simulink model "Models"  (R2022a)
settings: Solver=VariableStepAuto  StartTime=0.0  StopTime=15  RelTol=1e-6
settings Model: Creator=derekyu  LastModifiedBy=derekyu

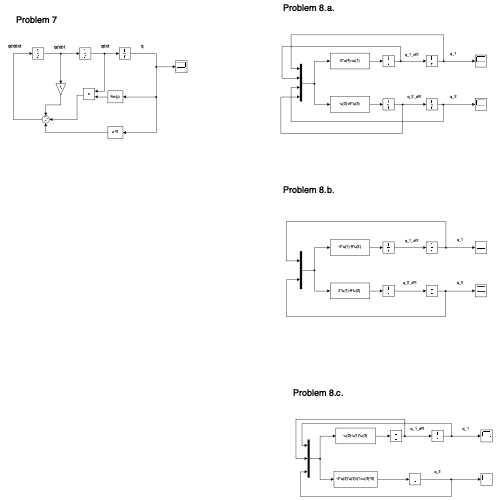
[thumbnail: Simulink's stored preview of the top-level diagram]
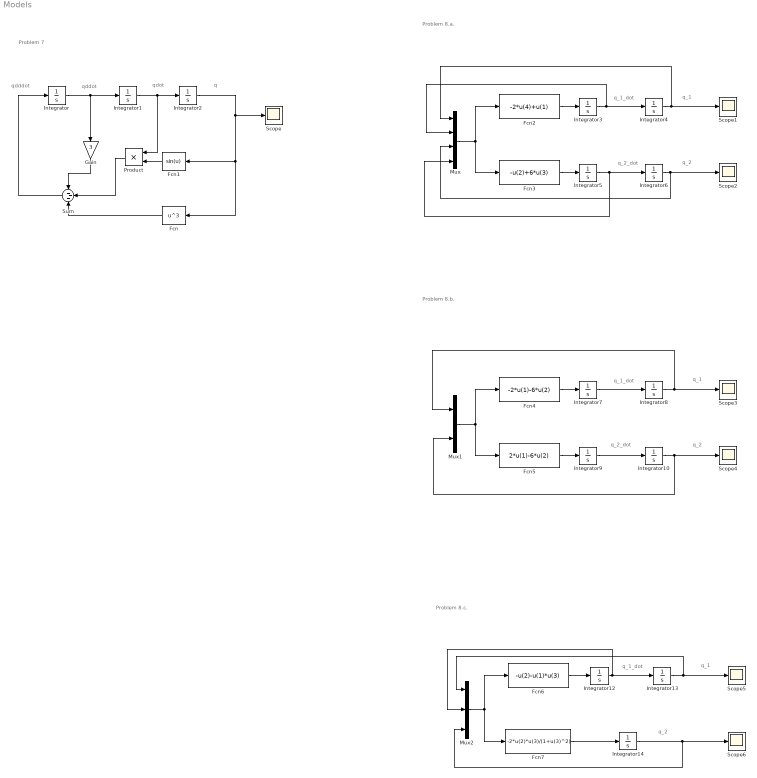
== system Models ==
  note: q_1_dot
  note: qdddot
  note: Problem 7
  note: qddot
  note: qdot
  note: q
  note: Problem 8.a.
  note: q_1
  note: q_2_dot
  note: q_2
  note: Problem 8.b.
  note: q_2
  note: q_1
  note: q_2_dot
  note: q_1_dot
  note: Problem 8.c.
  note: q_2
  note: q_1
  note: q_1_dot
  Fcn : Fcn  Expr=u^3
  Fcn1 : Fcn  Expr=sin(u)
  Fcn2 : Fcn  Expr=-2*u(4)+u(1)
  Fcn3 : Fcn  Expr=-u(2)+6*u(3)
  Fcn4 : Fcn  Expr=-2*u(1)-6*u(2)
  Fcn5 : Fcn  Expr=2*u(1)-6*u(2)
  Fcn6 : Fcn  Expr=-u(2)-u(1)*u(3)
  Fcn7 : Fcn  Expr=-2*u(2)*u(3)/(1+u(3)^2)
  Gain : Gain  Gain=3
  Integrator{,1,3,5,7,9,12} (7 alike) : Integrator
  Integrator{2,4,6,8,10,13..14} (7 alike) : Integrator  InitialCondition=1
  Mux : Mux
  Mux1 : Mux  Inputs=2
  Mux2 : Mux  Inputs=3
  Product : Product
  Scope{,1..6} (7 alike) : Scope
  Sum : Sum  Inputs=---
  wires:
  Integrator/1 -> Integrator1/1, Gain/1
  Integrator1/1 -> Product/1, Integrator2/1
  Sum/1 -> Integrator/1
  Integrator2/1 -> Fcn/1, Fcn1/1, Scope/1
  Fcn/1 -> Sum/3
  Fcn1/1 -> Product/2
  Product/1 -> Sum/2
  Gain/1 -> Sum/1
  Fcn2/1 -> Integrator3/1
  Integrator3/1 -> Integrator4/1, Mux/2
  Integrator4/1 -> Mux/1, Scope1/1
  Fcn3/1 -> Integrator5/1
  Integrator5/1 -> Mux/4, Integrator6/1
  Integrator6/1 -> Mux/3, Scope2/1
  Mux/1 -> Fcn2/1, Fcn3/1
  Integrator10/1 -> Mux1/2, Scope4/1
  Fcn4/1 -> Integrator7/1
  Mux1/1 -> Fcn4/1, Fcn5/1
  Integrator9/1 -> Integrator10/1
  Integrator7/1 -> Integrator8/1
  Fcn5/1 -> Integrator9/1
  Integrator8/1 -> Mux1/1, Scope3/1
  Integrator12/1 -> Mux2/2, Integrator13/1
  Mux2/1 -> Fcn6/1, Fcn7/1
  Integrator14/1 -> Mux2/3, Scope6/1
  Fcn7/1 -> Integrator14/1
  Fcn6/1 -> Integrator12/1
  Integrator13/1 -> Mux2/1, Scope5/1
